simulink model "motor_controle_velocidade_PI"  (R2019b)
settings: Solver=VariableStepAuto  StartTime=0.0  StopTime=7  RelTol=1e-3
settings Model: Creator=fernandopassold  LastModifiedBy=fernandopassold

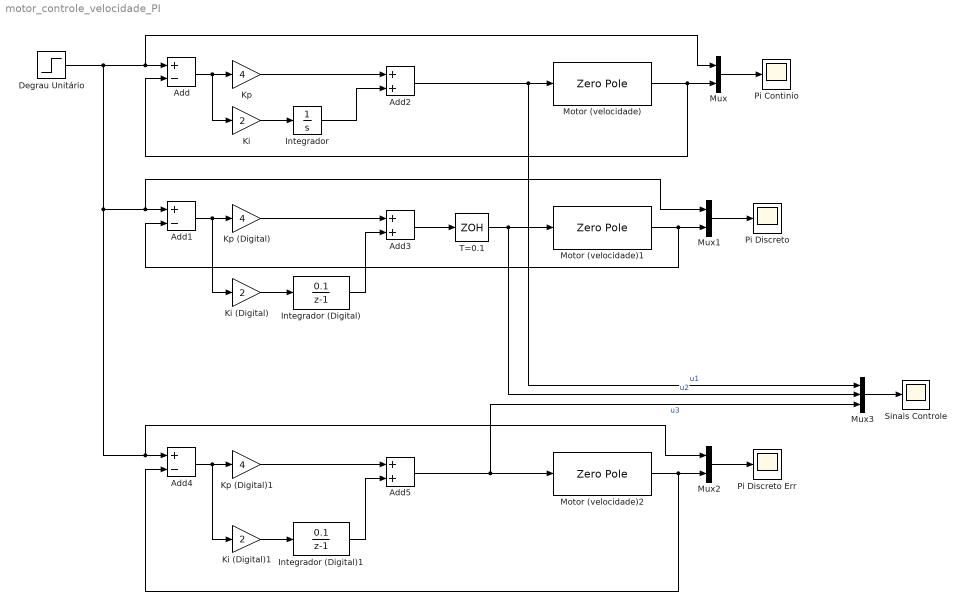
== system motor_controle_velocidade_PI ==
  Add : Sum  Inputs=+-
  Add1 : Sum  Inputs=+-
  Add2 : Sum
  Add3 : Sum
  Add4 : Sum  Inputs=+-
  Add5 : Sum
  Degrau Unitário : Step  SampleTime=0
  Integrador : Integrator
  Integrador (Digital) : DiscreteTransferFcn  Numerator=[0.1]  Denominator=[1 -1]  SampleTime=0.1
  Integrador (Digital)1 : DiscreteTransferFcn  Numerator=[0.1]  Denominator=[1 -1]  SampleTime=0.1
  Ki : Gain  Gain=2
  Ki (Digital) : Gain  Gain=2
  Ki (Digital)1 : Gain  Gain=2
  Kp : Gain  Gain=4
  Kp (Digital) : Gain  Gain=4
  Kp (Digital)1 : Gain  Gain=4
  Motor (velocidade) : ZeroPole  Zeros=[]  Poles=[-2 -1/2]
  Motor (velocidade)1 : ZeroPole  Zeros=[]  Poles=[-2 -1/2]
  Motor (velocidade)2 : ZeroPole  Zeros=[]  Poles=[-2 -1/2]
  Mux : Mux  Inputs=2
  Mux1 : Mux  Inputs=2
  Mux2 : Mux  Inputs=2
  Mux3 : Mux  Inputs=3
  Pi Continio : Scope
  Pi Discreto : Scope
  Pi Discreto Err : Scope
  Sinais Controle : Scope
  T=0.1 : ZeroOrderHold  SampleTime=0.1
  wires:
  Add/1 -> Ki/1, Kp/1
  Motor (velocidade)/1 -> Mux/2, Add/2
  Mux/1 -> Pi Continio/1
  Motor (velocidade)1/1 -> Add1/2, Mux1/2
  Add1/1 -> Ki (Digital)/1, Kp (Digital)/1
  Mux1/1 -> Pi Discreto/1
  T=0.1/1 -> Mux3/2, Motor (velocidade)1/1  "u2"
  Ki/1 -> Integrador/1
  Add2/1 -> Mux3/1, Motor (velocidade)/1  "u1"
  Kp/1 -> Add2/1
  Integrador/1 -> Add2/2
  Ki (Digital)/1 -> Integrador (Digital)/1
  Kp (Digital)/1 -> Add3/1
  Integrador (Digital)/1 -> Add3/2
  Add3/1 -> T=0.1/1
  Ki (Digital)1/1 -> Integrador (Digital)1/1
  Motor (velocidade)2/1 -> Add4/2, Mux2/2
  Integrador (Digital)1/1 -> Add5/2
  Degrau Unitário/1 -> Mux2/1, Add4/1, Mux1/1, Add1/1, Mux/1, Add/1
  Add4/1 -> Ki (Digital)1/1, Kp (Digital)1/1
  Mux2/1 -> Pi Discreto Err/1
  Kp (Digital)1/1 -> Add5/1
  Add5/1 -> Mux3/3, Motor (velocidade)2/1  "u3"
  Mux3/1 -> Sinais Controle/1
